simulink model "Ex6Tarefa6"  (R2020a)
settings: Solver=VariableStepAuto  StartTime=0.0  StopTime=0.1  RelTol=1e-3
libraries: simulink x2
settings Model: Creator=Joao Loureiro  LastModifiedBy=Joao Loureiro

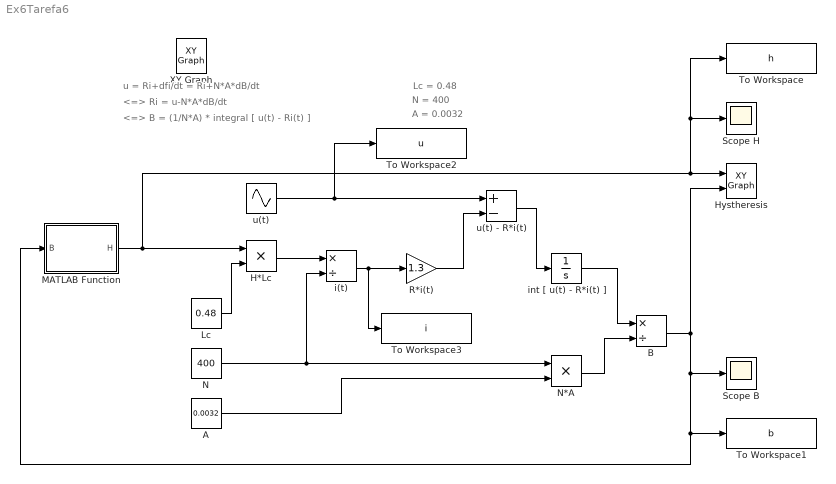
== system Ex6Tarefa6 ==
  note: A = 0.0032
  note: N = 400
  note: Lc = 0.48
  note: <=> B = (1/N*A) * integral [ u(t) - Ri(t) ]
  note: <=> Ri = u-N*A*dB/dt
  note: u = Ri+dfi/dt = Ri+N*A*dB/dt
  A : Constant  Value=0.0032
  B : Product  Inputs=*/
  H*Lc : Product
  Hystheresis : simulink/Sinks/XY Graph  xmin=0  xmax=1000  ymin=0  ymax=2  st=0.001
  Lc : Constant  Value=0.48
  MATLAB Function : MATLAB Function  TreatAsAtomicUnit=on
  N : Constant  Value=400
  N*A : Product
  R*i(t) : Gain  Gain=1.3
  Scope B : Scope
  Scope H : Scope
  To Workspace : ToWorkspace  VariableName=h  SaveFormat=Timeseries  SampleTime=-1
  To Workspace1 : ToWorkspace  VariableName=b  SaveFormat=Timeseries  SampleTime=-1
  To Workspace2 : ToWorkspace  VariableName=u  SaveFormat=Timeseries  SampleTime=-1
  To Workspace3 : ToWorkspace  VariableName=i  SaveFormat=Timeseries  SampleTime=-1
  i(t) : Product  Inputs=*/
  int [ u(t) - R*i(t) ] : Integrator
  u(t) : Sin  Amplitude=220*sqrt(2)  Frequency=50*2*pi  SampleTime=0
  u(t) - R*i(t) : Sum  Inputs=+-
  XY Graph : simulink/Sinks/XY Graph  IOType=viewer  xmin=-1  xmax=1  ymin=-1  ymax=1  st=-1
  wires:
  i(t)/1 -> To Workspace3/1, R*i(t)/1
  u(t)/1 -> u(t) - R*i(t)/1, To Workspace2/1
  R*i(t)/1 -> u(t) - R*i(t)/2
  u(t) - R*i(t)/1 -> int [ u(t) - R*i(t) ]/1
  N/1 -> N*A/1, i(t)/2
  A/1 -> N*A/2
  int [ u(t) - R*i(t) ]/1 -> B/1
  N*A/1 -> B/2
  MATLAB Function/1(H) -> To Workspace/1, Scope H/1, Hystheresis/1, H*Lc/1
  H*Lc/1 -> i(t)/1
  Lc/1 -> H*Lc/2
  B/1 -> Hystheresis/2, MATLAB Function/1(B), To Workspace1/1, Scope B/1

== matlab function Ex6Tarefa6/MATLAB Function ==
  data: B input; H output
function H = ObtemH(B)

m1 = 0.003143;
    b1 = 0;
    %upper_elbow
    m2 = 0.001;
    b2 = 0.75;
    %lower_elbow
    m3 = 0.001;
    b3 =-0.75;
    %saturation_upper
    m4 = 0;
    b4 = 1.75;
    %saturation_lower
    m5 = 0.0002;
    b5 = -1.03;
    if B >= -1.1 && B <= 1.1
        H = B/m1;
    else
        H = 0;
    end
    if B >= 1.1 && B <= 1.75
        H = (B - b2)/m2;
    end
    if B >= 1.75
        H = (B - 1.5833333)/(1.6*(10^-4));
    end
    if B <= -1.75
        H = (B + 1.5833333)/(1.6*(10^-4));
    end
    if B <= -1.1 && B >= -1.75
       H = (B + b2)/m2;
    end
%
%     if B <= -1.75
%         H = (B + 1.7)/(0.00005);
%     end
%
%     if B >= -1.75 && B <= 1.1
%         H = (B + b2 )/m2;
%     end

end
